simulink library "hvs_framelib_gen"  (R2016a)
settings: Solver=ode45  StartTime=0.0  StopTime=10.0  RelTol=1e-3
undefined symbols (not defined in the file): API4dcac_efficiency, API5dcac_efficiency, aux_power_flag, dcdc_effmap, dcdc_effmap_cooltemp_3rdD, dcdc_effmap_cur_2ndD, dcdc_effmap_vlt_1stD
libraries: Electrical_to_Mechanical_gen x6, Electrical_converter x2, Electrical_to_Thermal_gen x1, Electrical_charger x1, Powernet x1, ePTO x1, simulink x1
settings Model: Creator=krishs1  LastModifiedBy=krishs1
settings DataIOCC: LimitDataPoints=on
settings DebuggingCC: AllowSymbolicDim=off

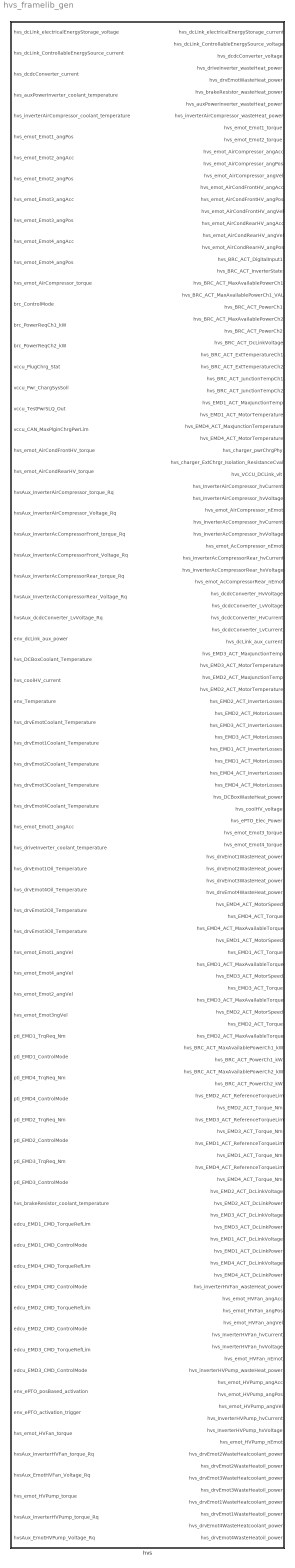
== system hvs_framelib_gen ==
  hvs : Subsystem

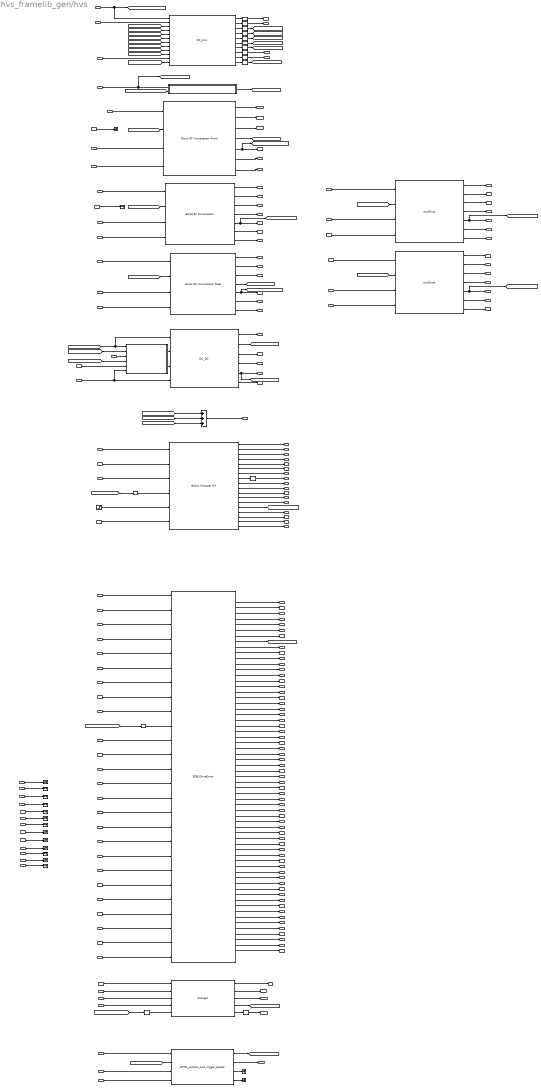
== system hvs_framelib_gen/hvs ==
  hvs_dcLink_electricalEnergyStorage_voltage : Inport
  hvs_dcLink_ControllableEnergySource_current : Inport  Port=2
  hvs_dcdcConverter_current : Inport  Port=3
  hvs_auxPowerInverter_coolant_temperature : Inport  Port=4
  hvs_inverterAirCompressor_coolant_temperature : Inport  Port=5
  hvs_emot_Emot1_angPos : Inport  Port=6
  hvs_emot_Emot2_angAcc : Inport  Port=7
  hvs_emot_Emot2_angPos : Inport  Port=8
  hvs_emot_Emot3_angAcc : Inport  Port=9
  hvs_emot_Emot3_angPos : Inport  Port=10
  hvs_emot_Emot4_angAcc : Inport  Port=11
  hvs_emot_Emot4_angPos : Inport  Port=12
  hvs_emot_AirCompressor_torque : Inport  Port=13
  brc_ControlMode : Inport  Port=14
  brc_PowerReqCh1_kW : Inport  Port=15
  brc_PowerReqCh2_kW : Inport  Port=16
  vccu_PlugChrg_Stat : Inport  Port=17
  vccu_Pwr_ChargSysSoll : Inport  Port=18
  vccu_TestPwrSLQ_Out : Inport  Port=19
  vccu_CAN_MaxPlginChrgPwrLim : Inport  Port=20
  hvs_emot_AirCondFrontHV_torque : Inport  Port=21
  hvs_emot_AirCondRearHV_torque : Inport  Port=22
  hvsAux_InverterAirCompressor_torque_Rq : Inport  Port=23
  hvsAux_InverterAirCompressor_Voltage_Rq : Inport  Port=24
  hvsAux_InverterAcCompressorFront_torque_Rq : Inport  Port=25
  hvsAux_InverterAcCompressorFront_Voltage_Rq : Inport  Port=26
  hvsAux_InverterAcCompressorRear_torque_Rq : Inport  Port=27
  hvsAux_InverterAcCompressorRear_Voltage_Rq : Inport  Port=28
  hvsAux_dcdcConverter_LvVoltage_Rq : Inport  Port=29
  env_dcLink_aux_power : Inport  Port=30
  hvs_DCBoxCoolant_Temperature : Inport  Port=31
  hvs_coolHV_current : Inport  Port=32
  env_Temperature : Inport  Port=33
  hvs_drvEmotCoolant_Temperature : Inport  Port=34
  hvs_drvEmot1Coolant_Temperature : Inport  Port=35
  hvs_drvEmot2Coolant_Temperature : Inport  Port=36
  hvs_drvEmot3Coolant_Temperature : Inport  Port=37
  hvs_drvEmot4Coolant_Temperature : Inport  Port=38
  hvs_emot_Emot1_angAcc : Inport  Port=39
  hvs_driveInverter_coolant_temperature : Inport  Port=40
  hvs_drvEmot1Oil_Temperature : Inport  Port=41
  hvs_drvEmot4Oil_Temperature : Inport  Port=42
  hvs_drvEmot2Oil_Temperature : Inport  Port=43
  hvs_drvEmot3Oil_Temperature : Inport  Port=44
  hvs_emot_Emot1_angVel : Inport  Port=45
  hvs_emot_Emot4_angVel : Inport  Port=46
  hvs_emot_Emot2_angVel : Inport  Port=47
  hvs_emot_Emot3ngVel : Inport  Port=48
  pti_EMD1_TrqReq_Nm : Inport  Port=49
  pti_EMD1_ControlMode : Inport  Port=50
  pti_EMD4_TrqReq_Nm : Inport  Port=51
  pti_EMD4_ControlMode : Inport  Port=52
  pti_EMD2_TrqReq_Nm : Inport  Port=53
  pti_EMD2_ControlMode : Inport  Port=54
  pti_EMD3_TrqReq_Nm : Inport  Port=55
  pti_EMD3_ControlMode : Inport  Port=56
  hvs_brakeResistor_coolant_temperature : Inport  Port=57
  edcu_EMD1_CMD_TorqueRefLim : Inport  Port=58
  edcu_EMD1_CMD_ControlMode : Inport  Port=59
  edcu_EMD4_CMD_TorqueRefLim : Inport  Port=60
  edcu_EMD4_CMD_ControlMode : Inport  Port=61
  edcu_EMD2_CMD_TorqueRefLim : Inport  Port=62
  edcu_EMD2_CMD_ControlMode : Inport  Port=63
  edcu_EMD3_CMD_TorqueRefLim : Inport  Port=64
  edcu_EMD3_CMD_ControlMode : Inport  Port=65
  env_ePTO_posBased_activation : Inport  Port=66
  env_ePTO_activation_trigger : Inport  Port=67
  hvs_emot_HVFan_torque : Inport  Port=68
  hvsAux_InverterHVFan_torque_Rq : Inport  Port=69
  hvsAux_EmotHVFan_Voltage_Rq : Inport  Port=70
  hvs_emot_HVPump_torque : Inport  Port=71
  hvsAux_InverterHVPump_torque_Rq : Inport  Port=72
  hvsAux_EmotHVPump_Voltage_Rq : Inport  Port=73
  Brake Chopper RX : Electrical_to_Thermal_gen/Brake Chopper RX
  Charger : Electrical_charger/Charger
  DC_DC : Electrical_converter/DC_DC
  DC_Link : Powernet/DC_Link
  EDB_DriveEmot : Electrical_to_Mechanical_gen/EDB_DriveEmot
  Emot AC Compressor Front : Electrical_to_Mechanical_gen/Emot AC Compressor Front
  Emot AC Compressor Rear : Electrical_to_Mechanical_gen/Emot AC Compressor Rear
  Emot Air Compressor : Electrical_to_Mechanical_gen/Emot Air Compressor
  Emotor Hv Fan : Electrical_to_Mechanical_gen/auxEmot  auxEmot_nTab_3rdD=emot_HVFan_nTab_3rdD  auxEmot_trqTab_2ndD=emot_HVFan_trqTab_2ndD  auxEmot_vltTab_1stD=emot_HVFan_vltTab_1stD  auxEmot_pwrAC=emot_HVFan_pwrAC  APIefficiency=1/API4dcac_efficiency  auxEmot_inertia=emot_HVFan_inertia  auxEmot_Tau=emot_HVFan_Tau  AWR_InvStError=0  auxEmot_power=0  aux_power_state=0
  Emotor Hv Pump : Electrical_to_Mechanical_gen/auxEmot  auxEmot_nTab_3rdD=emot_HVPump_nTab_3rdD  auxEmot_trqTab_2ndD=emot_HVPump_trqTab_2ndD  auxEmot_vltTab_1stD=emot_HVPump_vltTab_1stD  auxEmot_pwrAC=emot_HVPump_pwrAC  APIefficiency=1/API5dcac_efficiency  auxEmot_inertia=emot_HVPump_inertia  auxEmot_Tau=emot_HVPump_Tau  AWR_InvStError=0  auxEmot_power=0  aux_power_state=0
  HVFreigabeHW2_SiRelay_D : Step  Time=5.502
  Process : Subsystem
  Reshape{,1..8,11..12,14..17} (15 alike) : Reshape
  Sum8 : Sum  Inputs=+++  SaturateOnIntegerOverflow=on  InputSameDT=on  OutDataTypeStr=Inherit: Same as first input
  Terminator{,1..16} (17 alike) : Terminator
  ePTO_position_and_trigger_based : ePTO/ePTO_position_and_trigger_based
  sub_env_aux : Subsystem
  hvs_dcLink_electricalEnergyStorage_current : Outport
  hvs_dcLink_ControllableEnergySource_voltage : Outport  Port=2
  hvs_dcdcConverter_voltage : Outport  Port=3
  hvs_driveInverter_wasteHeat_power : Outport  Port=4
  hvs_drvEmotWasteHeat_power : Outport  Port=5
  hvs_brakeResistor_wasteHeat_power : Outport  Port=6
  hvs_auxPowerInverter_wasteHeat_power : Outport  Port=7
  hvs_inverterAirCompressor_wasteHeat_power : Outport  Port=8
  hvs_emot_Emot1_torque : Outport  Port=9
  hvs_emot_Emot2_torque : Outport  Port=10
  hvs_emot_AirCompressor_angAcc : Outport  Port=11
  hvs_emot_AirCompressor_angPos : Outport  Port=12
  hvs_emot_AirCompressor_angVel : Outport  Port=13
  hvs_emot_AirCondFrontHV_angAcc : Outport  Port=14
  hvs_emot_AirCondFrontHV_angPos : Outport  Port=15
  hvs_emot_AirCondFrontHV_angVel : Outport  Port=16
  hvs_emot_AirCondRearHV_angAcc : Outport  Port=17
  hvs_emot_AirCondRearHV_angVel : Outport  Port=18
  hvs_emot_AirCondRearHV_angPos : Outport  Port=19
  hvs_BRC_ACT_DigitalInput1 : Outport  Port=20
  hvs_BRC_ACT_InverterState : Outport  Port=21
  hvs_BRC_ACT_MaxAvailablePowerCh1 : Outport  Port=22
  hvs_BRC_ACT_MaxAvailablePowerCh1_VAL : Outport  Port=23
  hvs_BRC_ACT_PowerCh1 : Outport  Port=24
  hvs_BRC_ACT_MaxAvailablePowerCh2 : Outport  Port=25
  hvs_BRC_ACT_PowerCh2 : Outport  Port=26
  hvs_BRC_ACT_DcLinkVoltage : Outport  Port=27
  hvs_BRC_ACT_ExtTemperatureCh1 : Outport  Port=28
  hvs_BRC_ACT_ExtTemperatureCh2 : Outport  Port=29
  hvs_BRC_ACT_JunctionTempCh1 : Outport  Port=30
  hvs_BRC_ACT_JunctionTempCh2 : Outport  Port=31
  hvs_EMD1_ACT_MaxJunctionTemp : Outport  Port=32
  hvs_EMD1_ACT_MotorTemperature : Outport  Port=33
  hvs_EMD4_ACT_MaxJunctionTemperature : Outport  Port=34
  hvs_EMD4_ACT_MotorTemperature : Outport  Port=35
  hvs_charger_pwrChrgPhy : Outport  Port=36
  hvs_charger_ExtChrgr_Isolation_ResistanceCval : Outport  Port=37
  hvs_VCCU_DCLink_vlt : Outport  Port=38
  hvs_InverterAirCompressor_hvCurrent : Outport  Port=39
  hvs_InverterAirCompressor_hvVoltage : Outport  Port=40
  hvs_emot_AirCompressor_nEmot : Outport  Port=41
  hvs_InverterAcCompressor_hvCurrent : Outport  Port=42
  hvs_InverterAcCompressor_hvVoltage : Outport  Port=43
  hvs_emot_AcCompressor_nEmot : Outport  Port=44
  hvs_InverterAcCompressorRear_hvCurrent : Outport  Port=45
  hvs_InverterAcCompressorRear_hvVoltage : Outport  Port=46
  hvs_emot_AcCompressorRear_nEmot : Outport  Port=47
  hvs_dcdcConverter_HvVoltage : Outport  Port=48
  hvs_dcdcConverter_LvVoltage : Outport  Port=49
  hvs_dcdcConverter_HvCurrent : Outport  Port=50
  hvs_dcdcConverter_LvCurrent : Outport  Port=51
  hvs_dcLink_aux_current : Outport  Port=52
  hvs_EMD3_ACT_MaxJunctionTemp : Outport  Port=53
  hvs_EMD3_ACT_MotorTemperature : Outport  Port=54
  hvs_EMD2_ACT_MaxJunctionTemp : Outport  Port=55
  hvs_EMD2_ACT_MotorTemperature : Outport  Port=56
  hvs_EMD2_ACT_InverterLosses : Outport  Port=57
  hvs_EMD2_ACT_MotorLosses : Outport  Port=58
  hvs_EMD3_ACT_InverterLosses : Outport  Port=59
  hvs_EMD3_ACT_MotorLosses : Outport  Port=60
  hvs_EMD1_ACT_InverterLosses : Outport  Port=61
  hvs_EMD1_ACT_MotorLosses : Outport  Port=62
  hvs_EMD4_ACT_InverterLosses : Outport  Port=63
  hvs_EMD4_ACT_MotorLosses : Outport  Port=64
  hvs_DCBoxWasteHeat_power : Outport  Port=65
  hvs_coolHV_voltage : Outport  Port=66
  hvs_ePTO_Elec_Power : Outport  Port=67
  hvs_emot_Emot3_torque : Outport  Port=68
  hvs_emot_Emot4_torque : Outport  Port=69
  hvs_drvEmot1WasteHeat_power : Outport  Port=70
  hvs_drvEmot2WasteHeat_power : Outport  Port=71
  hvs_drvEmot3WasteHeat_power : Outport  Port=72
  hvs_drvEmot4WasteHeat_power : Outport  Port=73
  hvs_EMD4_ACT_MotorSpeed : Outport  Port=74
  hvs_EMD4_ACT_Torque : Outport  Port=75
  hvs_EMD4_ACT_MaxAvailableTorque : Outport  Port=76
  hvs_EMD1_ACT_MotorSpeed : Outport  Port=77
  hvs_EMD1_ACT_Torque : Outport  Port=78
  hvs_EMD1_ACT_MaxAvailableTorque : Outport  Port=79
  hvs_EMD3_ACT_MotorSpeed : Outport  Port=80
  hvs_EMD3_ACT_Torque : Outport  Port=81
  hvs_EMD3_ACT_MaxAvailableTorque : Outport  Port=82
  hvs_EMD2_ACT_MotorSpeed : Outport  Port=83
  hvs_EMD2_ACT_Torque : Outport  Port=84
  hvs_EMD2_ACT_MaxAvailableTorque : Outport  Port=85
  hvs_BRC_ACT_MaxAvailablePowerCh1_kW : Outport  Port=86
  hvs_BRC_ACT_PowerCh1_kW : Outport  Port=87
  hvs_BRC_ACT_MaxAvailablePowerCh2_kW : Outport  Port=88
  hvs_BRC_ACT_PowerCh2_kW : Outport  Port=89
  hvs_EMD2_ACT_ReferenceTorqueLim : Outport  Port=90
  hvs_EMD2_ACT_Torque_Nm : Outport  Port=91
  hvs_EMD3_ACT_ReferenceTorqueLim : Outport  Port=92
  hvs_EMD3_ACT_Torque_Nm : Outport  Port=93
  hvs_EMD1_ACT_ReferenceTorqueLim : Outport  Port=94
  hvs_EMD1_ACT_Torque_Nm : Outport  Port=95
  hvs_EMD4_ACT_ReferenceTorqueLim : Outport  Port=96
  hvs_EMD4_ACT_Torque_Nm : Outport  Port=97
  hvs_EMD2_ACT_DcLinkVoltage : Outport  Port=98
  hvs_EMD2_ACT_DcLinkPower : Outport  Port=99
  hvs_EMD3_ACT_DcLinkVoltage : Outport  Port=100
  hvs_EMD3_ACT_DcLinkPower : Outport  Port=101
  hvs_EMD1_ACT_DcLinkVoltage : Outport  Port=102
  hvs_EMD1_ACT_DcLinkPower : Outport  Port=103
  hvs_EMD4_ACT_DcLinkVoltage : Outport  Port=104
  hvs_EMD4_ACT_DcLinkPower : Outport  Port=105
  hvs_inverterHVFan_wasteHeat_power : Outport  Port=106
  hvs_emot_HVFan_angAcc : Outport  Port=107
  hvs_emot_HVFan_angPos : Outport  Port=108
  hvs_emot_HVFan_angVel : Outport  Port=109
  hvs_InverterHVFan_hvCurrent : Outport  Port=110
  hvs_InverterHVFan_hvVoltage : Outport  Port=111
  hvs_emot_HVFan_nEmot : Outport  Port=112
  hvs_inverterHVPump_wasteHeat_power : Outport  Port=113
  hvs_emot_HVPump_angAcc : Outport  Port=114
  hvs_emot_HVPump_angPos : Outport  Port=115
  hvs_emot_HVPump_angVel : Outport  Port=116
  hvs_InverterHVPump_hvCurrent : Outport  Port=117
  hvs_InverterHVPump_hvVoltage : Outport  Port=118
  hvs_emot_HVPump_nEmot : Outport  Port=119
  hvs_drvEmot2WasteHeatcoolant_power : Outport  Port=120
  hvs_drvEmot2WasteHeatoil_power : Outport  Port=121
  hvs_drvEmot3WasteHeatcoolant_power : Outport  Port=122
  hvs_drvEmot3WasteHeatoil_power : Outport  Port=123
  hvs_drvEmot1WasteHeatcoolant_power : Outport  Port=124
  hvs_drvEmot1WasteHeatoil_power : Outport  Port=125
  hvs_drvEmot4WasteHeatcoolant_power : Outport  Port=126
  hvs_drvEmot4WasteHeatoil_power : Outport  Port=127
  wires:
  EDB_DriveEmot/29 -> hvs_EMD4_ACT_Torque/1
  EDB_DriveEmot/28 -> hvs_EMD4_ACT_MotorSpeed/1
  EDB_DriveEmot/27 -> hvs_drvEmot4WasteHeat_power/1
  EDB_DriveEmot/26 -> hvs_drvEmot3WasteHeat_power/1
  EDB_DriveEmot/8 -> [hvs_dcLink_drive_emot_current]
  hvs_drvEmot4Coolant_Temperature/1 -> Terminator14/1
  hvs_drvEmot3Coolant_Temperature/1 -> Terminator13/1
  hvs_drvEmot2Coolant_Temperature/1 -> Terminator12/1
  hvs_drvEmot1Coolant_Temperature/1 -> Terminator11/1
  EDB_DriveEmot/25 -> hvs_drvEmot2WasteHeat_power/1
  EDB_DriveEmot/24 -> hvs_drvEmot1WasteHeat_power/1
  hvs_emot_Emot4_angPos/1 -> Terminator10/1
  hvs_emot_Emot4_angAcc/1 -> Terminator9/1
  hvs_emot_Emot3_angPos/1 -> Terminator8/1
  hvs_emot_Emot3_angAcc/1 -> Terminator6/1
  Process/2(hvs_dcdcConv_current1) -> DC_DC/3
  Process/1(dcdc_conv_eff) -> DC_DC/2
  hvs_dcdcConverter_current/1 -> Process/5(hvs_dcdcConv_current)
  [dcLink_aux_power] -> Process/4(dcLink_aux_power)  "dcLink_aux_power"
  hvs_drvEmotCoolant_Temperature/1 -> Process/3(hvs_drvEmotCoolant_Temperature)
  [hvs_dcdc_current] -> Process/2(hvs_dcdc_HvCurrent)  "hvs_dcdc_HvCurrent"
  [hvs_dcLink_ePTO_current] -> DC_Link/12
  [hvs_APIs_DCLink_vlt] -> ePTO_position_and_trigger_based/2
  ePTO_position_and_trigger_based/3 -> Terminator7/1
  ePTO_position_and_trigger_based/2 -> hvs_ePTO_Elec_Power/1
  ePTO_position_and_trigger_based/1 -> [hvs_dcLink_ePTO_current]
  DC_Link/10 -> Reshape17/1
  Reshape17/1 -> [hvs_ePTO_DCLink_vlt]
  env_Temperature/1 -> ePTO_position_and_trigger_based/1
  EDB_DriveEmot/23 -> hvs_emot_Emot4_torque/1
  EDB_DriveEmot/22 -> hvs_emot_Emot3_torque/1
  hvs_DCBoxCoolant_Temperature/1 -> Terminator4/1
  Charger/1 -> hvs_DCBoxWasteHeat_power/1  "hvs_DCBoxWasteHeat_power"
  hvsAux_dcdcConverter_LvVoltage_Rq/1 -> DC_DC/4, Process/6(hvsAux_dcdcConv_LvVoltage_Rq)  "hvsAux_dcdcConverter_LvVoltage_Rq"
  DC_Link/8 -> Reshape15/1
  [hvs_dcLink_electricalEnergyStorage_voltage] -> sub_env_aux/2(Nebenagg_voltage)
  sub_env_aux/1(dcLink_aux_current) -> [dcLink_aux_current]
  env_dcLink_aux_power/1 -> sub_env_aux/1(env_dcLink_aux_power), [dcLink_aux_power]
  [dcLink_aux_current] -> DC_Link/10
  Reshape12/1 -> hvs_VCCU_DCLink_vlt/1
  Reshape11/1 -> Charger/5
  Reshape7/1 -> hvs_BRC_ACT_DcLinkVoltage/1
  Reshape6/1 -> Brake Chopper RX/4
  Reshape5/1 -> [hvs_APIs_DCLink_vlt]
  Reshape4/1 -> [hvs_charger_DCLink_vlt]
  Reshape3/1 -> [hvs_inverter_drive_emot_voltage]
  Reshape2/1 -> [hvs_inverter_BrakeResistor_voltage]
  Reshape1/1 -> [hvs_dcdcConverter_voltage]
  Reshape/1 -> hvs_dcLink_electricalEnergyStorage_current/1
  [hvs_dcdc_current] -> DC_Link/3
  [hvs_DCL_wasteHeat_power] -> Sum8/3
  [hvs_API3_wasteHeat_power] -> Sum8/2
  [hvs_API1_wasteHeat_power] -> Sum8/1
  Sum8/1 -> hvs_auxPowerInverter_wasteHeat_power/1
  DC_DC/6 -> hvs_dcdcConverter_LvCurrent/1
  DC_DC/5 -> hvs_dcdcConverter_HvCurrent/1, [hvs_dcdc_current]
  DC_DC/4 -> hvs_dcdcConverter_LvVoltage/1
  DC_DC/3 -> hvs_dcdcConverter_HvVoltage/1
  DC_Link/3 -> Reshape1/1
  DC_DC/1 -> hvs_dcdcConverter_voltage/1
  DC_DC/2 -> [hvs_DCL_wasteHeat_power]
  [hvs_dcdcConverter_voltage] -> Process/1(hvs_dcdcConverter_voltage), DC_DC/1  "hvs_dcdcConverter_voltage"
  Emot AC Compressor Rear/4 -> [hvs_API3_wasteHeat_power]
  Emot AC Compressor Rear/5 -> hvs_InverterAcCompressorRear_hvCurrent/1, [hvs_InverterAcCompressorRear_hvCurrent]
  Emot AC Compressor Rear/6 -> hvs_InverterAcCompressorRear_hvVoltage/1
  Emot AC Compressor Rear/7 -> hvs_emot_AcCompressorRear_nEmot/1
  Emot AC Compressor Rear/2 -> hvs_emot_AirCondRearHV_angPos/1
  Emot AC Compressor Rear/3 -> hvs_emot_AirCondRearHV_angVel/1
  Emot AC Compressor Rear/1 -> hvs_emot_AirCondRearHV_angAcc/1
  hvsAux_InverterAcCompressorRear_Voltage_Rq/1 -> Emot AC Compressor Rear/4
  hvsAux_InverterAcCompressorRear_torque_Rq/1 -> Emot AC Compressor Rear/3
  [hvs_APIs_DCLink_vlt] -> Emot AC Compressor Rear/2
  hvs_emot_AirCondRearHV_torque/1 -> Emot AC Compressor Rear/1
  Emot AC Compressor Front/4 -> [hvs_API1_wasteHeat_power]
  Emot AC Compressor Front/6 -> hvs_InverterAcCompressor_hvVoltage/1
  Emot AC Compressor Front/7 -> hvs_emot_AcCompressor_nEmot/1
  Emot AC Compressor Front/3 -> hvs_emot_AirCondFrontHV_angVel/1
  Emot AC Compressor Front/2 -> hvs_emot_AirCondFrontHV_angPos/1
  Emot AC Compressor Front/1 -> hvs_emot_AirCondFrontHV_angAcc/1
  hvsAux_InverterAcCompressorFront_Voltage_Rq/1 -> Emot AC Compressor Front/4
  hvsAux_InverterAcCompressorFront_torque_Rq/1 -> Emot AC Compressor Front/3
  hvs_emot_AirCondFrontHV_torque/1 -> Emot AC Compressor Front/1
  [hvs_APIs_DCLink_vlt] -> Emot AC Compressor Front/2
  hvs_auxPowerInverter_coolant_temperature/1 -> Terminator5/1
  hvs_inverterAirCompressor_coolant_temperature/1 -> Terminator/1
  hvsAux_InverterAirCompressor_Voltage_Rq/1 -> Emot Air Compressor/4
  hvsAux_InverterAirCompressor_torque_Rq/1 -> Emot Air Compressor/3
  [hvs_APIs_DCLink_vlt] -> Emot Air Compressor/2
  DC_Link/7 -> Reshape5/1
  Emot Air Compressor/6 -> hvs_InverterAirCompressor_hvVoltage/1
  Emot Air Compressor/7 -> hvs_emot_AirCompressor_nEmot/1
  Emot Air Compressor/5 -> [hvs_emot_AirCompressor_emot_current], hvs_InverterAirCompressor_hvCurrent/1
  Emot Air Compressor/4 -> hvs_inverterAirCompressor_wasteHeat_power/1
  Emot Air Compressor/3 -> hvs_emot_AirCompressor_angVel/1
  Emot Air Compressor/2 -> hvs_emot_AirCompressor_angPos/1
  Emot Air Compressor/1 -> hvs_emot_AirCompressor_angAcc/1
  hvs_emot_AirCompressor_torque/1 -> Emot Air Compressor/1
  DC_Link/1 -> Reshape/1
  DC_Link/2 -> Reshape14/1
  hvs_dcLink_electricalEnergyStorage_voltage/1 -> [hvs_dcLink_electricalEnergyStorage_voltage], DC_Link/1
  hvs_dcLink_ControllableEnergySource_current/1 -> DC_Link/2
  DC_Link/4 -> Reshape2/1
  Brake Chopper RX/1 -> hvs_BRC_ACT_DigitalInput1/1
  Brake Chopper RX/2 -> hvs_BRC_ACT_InverterState/1
  Brake Chopper RX/3 -> hvs_BRC_ACT_MaxAvailablePowerCh1/1
  Brake Chopper RX/4 -> hvs_BRC_ACT_MaxAvailablePowerCh1_VAL/1
  Brake Chopper RX/5 -> hvs_BRC_ACT_PowerCh1/1
  Brake Chopper RX/6 -> hvs_BRC_ACT_MaxAvailablePowerCh2/1
  Brake Chopper RX/7 -> hvs_BRC_ACT_PowerCh2/1
  Brake Chopper RX/8 -> Reshape7/1
  Brake Chopper RX/9 -> hvs_BRC_ACT_ExtTemperatureCh1/1
  Brake Chopper RX/10 -> hvs_BRC_ACT_ExtTemperatureCh2/1
  Brake Chopper RX/11 -> hvs_BRC_ACT_JunctionTempCh1/1
  Brake Chopper RX/12 -> hvs_BRC_ACT_JunctionTempCh2/1
  [hvs_inverter_BrakeResistor_voltage] -> Reshape6/1
  DC_Link/5 -> Reshape3/1
  [hvs_dcLink_drive_emot_current] -> DC_Link/4
  [hvs_emot_AirCompressor_emot_current] -> DC_Link/5
  Brake Chopper RX/13 -> hvs_brakeResistor_wasteHeat_power/1
  Brake Chopper RX/14 -> [hvs_dcLink_BrakeResistor_current]
  [hvs_dcLink_BrakeResistor_current] -> DC_Link/6
  hvs_emot_Emot1_angPos/1 -> Terminator1/1
  hvs_emot_Emot2_angAcc/1 -> Terminator2/1
  hvs_emot_Emot2_angPos/1 -> Terminator3/1
  EDB_DriveEmot/13 -> hvs_emot_Emot2_torque/1
  EDB_DriveEmot/4 -> hvs_EMD1_ACT_MaxJunctionTemp/1
  EDB_DriveEmot/5 -> hvs_EMD1_ACT_MotorTemperature/1
  EDB_DriveEmot/6 -> hvs_EMD4_ACT_MaxJunctionTemperature/1
  EDB_DriveEmot/7 -> hvs_EMD4_ACT_MotorTemperature/1
  vccu_CAN_MaxPlginChrgPwrLim/1 -> Charger/4
  [hvs_charger_DCLink_vlt] -> Reshape11/1
  vccu_TestPwrSLQ_Out/1 -> Charger/3
  vccu_Pwr_ChargSysSoll/1 -> Charger/2
  vccu_PlugChrg_Stat/1 -> Charger/1
  Charger/2 -> hvs_charger_pwrChrgPhy/1
  Charger/3 -> hvs_charger_ExtChrgr_Isolation_ResistanceCval/1
  Charger/4 -> [hvs_dcLink_charger_current]
  [hvs_dcLink_charger_current] -> DC_Link/7
  DC_Link/6 -> Reshape4/1
  Charger/5 -> Reshape12/1
  Emot AC Compressor Front/5 -> [hvs_InverterAcCompressor_hvCurrent], hvs_InverterAcCompressor_hvCurrent/1
  [hvs_InverterAcCompressor_hvCurrent] -> DC_Link/8
  [hvs_InverterAcCompressorRear_hvCurrent] -> DC_Link/9
  EDB_DriveEmot/1 -> hvs_emot_Emot1_torque/1
  EDB_DriveEmot/2 -> hvs_driveInverter_wasteHeat_power/1
  EDB_DriveEmot/3 -> hvs_drvEmotWasteHeat_power/1
  EDB_DriveEmot/9 -> hvs_EMD3_ACT_MaxJunctionTemp/1
  EDB_DriveEmot/10 -> hvs_EMD3_ACT_MotorTemperature/1
  EDB_DriveEmot/11 -> hvs_EMD2_ACT_MaxJunctionTemp/1
  EDB_DriveEmot/12 -> hvs_EMD2_ACT_MotorTemperature/1
  EDB_DriveEmot/14 -> hvs_EMD2_ACT_InverterLosses/1
  EDB_DriveEmot/15 -> hvs_EMD2_ACT_MotorLosses/1
  EDB_DriveEmot/16 -> hvs_EMD3_ACT_InverterLosses/1
  EDB_DriveEmot/17 -> hvs_EMD3_ACT_MotorLosses/1
  EDB_DriveEmot/18 -> hvs_EMD1_ACT_InverterLosses/1
  EDB_DriveEmot/19 -> hvs_EMD1_ACT_MotorLosses/1
  EDB_DriveEmot/20 -> hvs_EMD4_ACT_InverterLosses/1
  EDB_DriveEmot/21 -> hvs_EMD4_ACT_MotorLosses/1
  Reshape14/1 -> hvs_dcLink_ControllableEnergySource_voltage/1
  Reshape15/1 -> hvs_dcLink_aux_current/1
  DC_Link/9 -> Reshape16/1
  Reshape16/1 -> hvs_coolHV_voltage/1
  hvs_coolHV_current/1 -> DC_Link/11
  hvs_emot_Emot1_angAcc/1 -> Terminator15/1
  EDB_DriveEmot/30 -> hvs_EMD4_ACT_MaxAvailableTorque/1
  EDB_DriveEmot/31 -> hvs_EMD1_ACT_MotorSpeed/1
  EDB_DriveEmot/32 -> hvs_EMD1_ACT_Torque/1
  EDB_DriveEmot/33 -> hvs_EMD1_ACT_MaxAvailableTorque/1
  EDB_DriveEmot/34 -> hvs_EMD3_ACT_MotorSpeed/1
  EDB_DriveEmot/35 -> hvs_EMD3_ACT_Torque/1
  EDB_DriveEmot/36 -> hvs_EMD3_ACT_MaxAvailableTorque/1
  EDB_DriveEmot/37 -> hvs_EMD2_ACT_MotorSpeed/1
  EDB_DriveEmot/38 -> hvs_EMD2_ACT_Torque/1
  EDB_DriveEmot/39 -> hvs_EMD2_ACT_MaxAvailableTorque/1
  EDB_DriveEmot/40 -> hvs_EMD2_ACT_ReferenceTorqueLim/1
  EDB_DriveEmot/41 -> hvs_EMD2_ACT_Torque_Nm/1
  hvs_driveInverter_coolant_temperature/1 -> EDB_DriveEmot/1
  hvs_drvEmot1Oil_Temperature/1 -> EDB_DriveEmot/2
  hvs_drvEmot4Oil_Temperature/1 -> EDB_DriveEmot/3
  hvs_drvEmot2Oil_Temperature/1 -> EDB_DriveEmot/4
  hvs_drvEmot3Oil_Temperature/1 -> EDB_DriveEmot/5
  hvs_emot_Emot1_angVel/1 -> EDB_DriveEmot/6
  hvs_emot_Emot4_angVel/1 -> EDB_DriveEmot/7
  hvs_emot_Emot2_angVel/1 -> EDB_DriveEmot/8
  hvs_emot_Emot3ngVel/1 -> EDB_DriveEmot/9
  [hvs_inverter_drive_emot_voltage] -> Reshape8/1
  Reshape8/1 -> EDB_DriveEmot/10
  HVFreigabeHW2_SiRelay_D/1 -> Brake Chopper RX/5
  pti_EMD1_TrqReq_Nm/1 -> EDB_DriveEmot/11
  pti_EMD1_ControlMode/1 -> EDB_DriveEmot/12
  pti_EMD4_TrqReq_Nm/1 -> EDB_DriveEmot/13
  pti_EMD4_ControlMode/1 -> EDB_DriveEmot/14
  pti_EMD2_TrqReq_Nm/1 -> EDB_DriveEmot/15
  pti_EMD2_ControlMode/1 -> EDB_DriveEmot/16
  pti_EMD3_TrqReq_Nm/1 -> EDB_DriveEmot/17
  pti_EMD3_ControlMode/1 -> EDB_DriveEmot/18
  brc_ControlMode/1 -> Brake Chopper RX/1
  brc_PowerReqCh1_kW/1 -> Brake Chopper RX/2
  brc_PowerReqCh2_kW/1 -> Brake Chopper RX/3
  hvs_brakeResistor_coolant_temperature/1 -> Brake Chopper RX/6
  Brake Chopper RX/15 -> hvs_BRC_ACT_MaxAvailablePowerCh1_kW/1
  Brake Chopper RX/16 -> hvs_BRC_ACT_PowerCh1_kW/1
  Brake Chopper RX/17 -> hvs_BRC_ACT_MaxAvailablePowerCh2_kW/1
  Brake Chopper RX/18 -> hvs_BRC_ACT_PowerCh2_kW/1
  EDB_DriveEmot/42 -> hvs_EMD3_ACT_ReferenceTorqueLim/1
  EDB_DriveEmot/44 -> hvs_EMD1_ACT_ReferenceTorqueLim/1
  EDB_DriveEmot/46 -> hvs_EMD4_ACT_ReferenceTorqueLim/1
  EDB_DriveEmot/47 -> hvs_EMD4_ACT_Torque_Nm/1
  EDB_DriveEmot/45 -> hvs_EMD1_ACT_Torque_Nm/1
  EDB_DriveEmot/48 -> hvs_EMD2_ACT_DcLinkVoltage/1
  EDB_DriveEmot/49 -> hvs_EMD2_ACT_DcLinkPower/1
  EDB_DriveEmot/50 -> hvs_EMD3_ACT_DcLinkVoltage/1
  EDB_DriveEmot/51 -> hvs_EMD3_ACT_DcLinkPower/1
  EDB_DriveEmot/52 -> hvs_EMD1_ACT_DcLinkVoltage/1
  EDB_DriveEmot/43 -> hvs_EMD3_ACT_Torque_Nm/1
  EDB_DriveEmot/54 -> hvs_EMD4_ACT_DcLinkVoltage/1
  EDB_DriveEmot/55 -> hvs_EMD4_ACT_DcLinkPower/1
  EDB_DriveEmot/53 -> hvs_EMD1_ACT_DcLinkPower/1
  edcu_EMD4_CMD_ControlMode/1 -> EDB_DriveEmot/22
  edcu_EMD2_CMD_ControlMode/1 -> EDB_DriveEmot/24
  edcu_EMD2_CMD_TorqueRefLim/1 -> EDB_DriveEmot/23
  edcu_EMD3_CMD_ControlMode/1 -> EDB_DriveEmot/26
  edcu_EMD3_CMD_TorqueRefLim/1 -> EDB_DriveEmot/25
  edcu_EMD4_CMD_TorqueRefLim/1 -> EDB_DriveEmot/21
  edcu_EMD1_CMD_TorqueRefLim/1 -> EDB_DriveEmot/19
  edcu_EMD1_CMD_ControlMode/1 -> EDB_DriveEmot/20
  ePTO_position_and_trigger_based/4 -> Terminator16/1
  env_ePTO_posBased_activation/1 -> ePTO_position_and_trigger_based/3
  env_ePTO_activation_trigger/1 -> ePTO_position_and_trigger_based/4
  hvsAux_EmotHVFan_Voltage_Rq/1 -> Emotor Hv Fan/4
  hvsAux_InverterHVFan_torque_Rq/1 -> Emotor Hv Fan/3
  [hvs_APIs_DCLink_vlt] -> Emotor Hv Fan/2
  Emotor Hv Fan/6 -> hvs_InverterHVFan_hvVoltage/1
  Emotor Hv Fan/7 -> hvs_emot_HVFan_nEmot/1
  Emotor Hv Fan/5 -> [hvs_emot_HVFan_emot_current], hvs_InverterHVFan_hvCurrent/1
  Emotor Hv Fan/4 -> hvs_inverterHVFan_wasteHeat_power/1
  Emotor Hv Fan/3 -> hvs_emot_HVFan_angVel/1
  Emotor Hv Fan/2 -> hvs_emot_HVFan_angPos/1
  Emotor Hv Fan/1 -> hvs_emot_HVFan_angAcc/1
  hvs_emot_HVFan_torque/1 -> Emotor Hv Fan/1
  [hvs_APIs_DCLink_vlt] -> Emotor Hv Pump/2
  hvsAux_EmotHVPump_Voltage_Rq/1 -> Emotor Hv Pump/4
  hvsAux_InverterHVPump_torque_Rq/1 -> Emotor Hv Pump/3
  hvs_emot_HVPump_torque/1 -> Emotor Hv Pump/1
  Emotor Hv Pump/6 -> hvs_InverterHVPump_hvVoltage/1
  Emotor Hv Pump/7 -> hvs_emot_HVPump_nEmot/1
  Emotor Hv Pump/5 -> [hvs_emot_HVPump_emot_current], hvs_InverterHVPump_hvCurrent/1
  Emotor Hv Pump/4 -> hvs_inverterHVPump_wasteHeat_power/1
  Emotor Hv Pump/3 -> hvs_emot_HVPump_angVel/1
  Emotor Hv Pump/2 -> hvs_emot_HVPump_angPos/1
  Emotor Hv Pump/1 -> hvs_emot_HVPump_angAcc/1
  EDB_DriveEmot/56 -> hvs_drvEmot2WasteHeatcoolant_power/1
  EDB_DriveEmot/57 -> hvs_drvEmot2WasteHeatoil_power/1
  EDB_DriveEmot/58 -> hvs_drvEmot3WasteHeatcoolant_power/1
  EDB_DriveEmot/59 -> hvs_drvEmot3WasteHeatoil_power/1
  EDB_DriveEmot/60 -> hvs_drvEmot1WasteHeatcoolant_power/1
  EDB_DriveEmot/61 -> hvs_drvEmot1WasteHeatoil_power/1
  EDB_DriveEmot/63 -> hvs_drvEmot4WasteHeatoil_power/1
  EDB_DriveEmot/62 -> hvs_drvEmot4WasteHeatcoolant_power/1

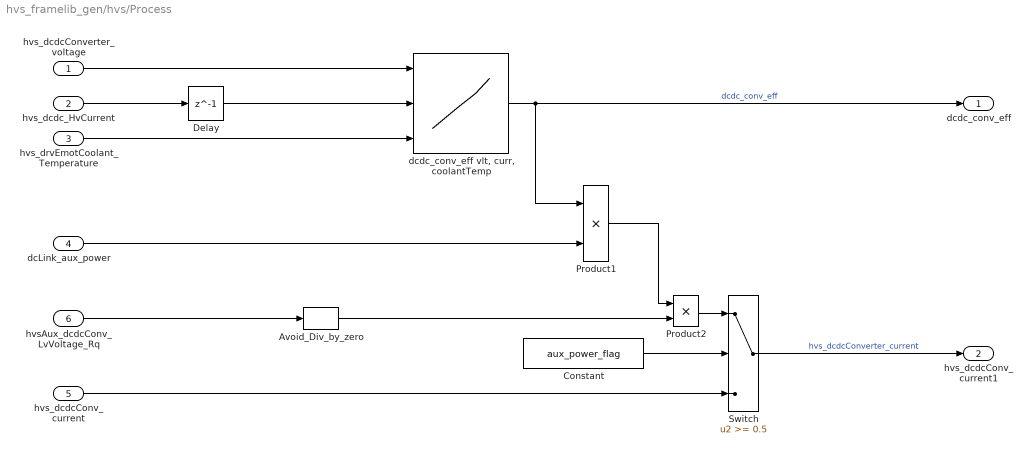
== system hvs_framelib_gen/hvs/Process ==
  hvs_dcdcConverter_voltage : Inport
  hvs_dcdc_HvCurrent : Inport  Port=2
  hvs_drvEmotCoolant_Temperature : Inport  Port=3
  dcLink_aux_power : Inport  Port=4
  hvs_dcdcConv_current : Inport  Port=5
  hvsAux_dcdcConv_LvVoltage_Rq : Inport  Port=6
  Avoid_Div_by_zero : Electrical_converter/DC_DC/Avoid_Div_by_zero
  Constant : Constant  Value=aux_power_flag
  Delay : Delay  DelayLength=1  InitialCondition=0
  Product1 : Product  Inputs=**  RndMeth=Zero
  Product2 : Product  Inputs=**  RndMeth=Zero
  Switch : Switch  Threshold=0.5
  "dcdc_conv_eff vlt, curr, coolantTemp" : Lookup_n-D  NumberOfTableDimensions=3  BreakpointsForDimension1=dcdc_effmap_vlt_1stD  BreakpointsForDimension2=dcdc_effmap_cur_2ndD  BreakpointsForDimension3=dcdc_effmap_cooltemp_3rdD  Table=dcdc_effmap  ExtrapMethod=Clip  RndMeth=Simplest  InputSameDT=on
  dcdc_conv_eff : Outport
  hvs_dcdcConv_current1 : Outport  Port=2
  wires:
  Delay/1 -> "dcdc_conv_eff vlt, curr, coolantTemp"/2
  hvs_dcdc_HvCurrent/1 -> Delay/1
  "dcdc_conv_eff vlt, curr, coolantTemp"/1 -> dcdc_conv_eff/1, Product1/1  "dcdc_conv_eff"
  Product2/1 -> Switch/1
  Product1/1 -> Product2/1
  hvs_dcdcConv_current/1 -> Switch/3
  Switch/1 -> hvs_dcdcConv_current1/1  "hvs_dcdcConverter_current"
  dcLink_aux_power/1 -> Product1/2
  Avoid_Div_by_zero/1 -> Product2/2
  Constant/1 -> Switch/2
  hvsAux_dcdcConv_LvVoltage_Rq/1 -> Avoid_Div_by_zero/1
  hvs_dcdcConverter_voltage/1 -> "dcdc_conv_eff vlt, curr, coolantTemp"/1
  hvs_drvEmotCoolant_Temperature/1 -> "dcdc_conv_eff vlt, curr, coolantTemp"/3

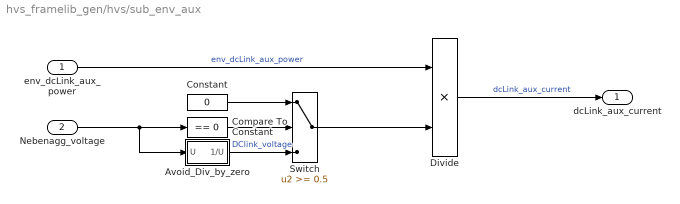
== system hvs_framelib_gen/hvs/sub_env_aux ==
  env_dcLink_aux_power : Inport
  Nebenagg_voltage : Inport  Port=2
  Avoid_Div_by_zero : Subsystem
  Compare To Constant : simulink/Logic and Bit Operations/Compare To Constant  relop===  const=0  OutDataTypeStr=boolean
  Constant : Constant  Value=0
  Divide : Product
  Switch : Switch  Threshold=0.5
  dcLink_aux_current : Outport
  wires:
  Divide/1 -> dcLink_aux_current/1  "dcLink_aux_current"
  Nebenagg_voltage/1 -> Avoid_Div_by_zero/1(U), Compare To Constant/1
  Avoid_Div_by_zero/1(1/U) -> Switch/3  "DClink_voltage"
  env_dcLink_aux_power/1 -> Divide/1  "env_dcLink_aux_power"
  Compare To Constant/1 -> Switch/2
  Constant/1 -> Switch/1
  Switch/1 -> Divide/2

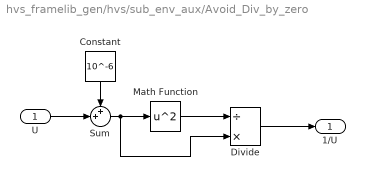
== system hvs_framelib_gen/hvs/sub_env_aux/Avoid_Div_by_zero ==
  U : Inport
  Constant : Constant  Value=10^-6
  Divide : Product  Inputs=/*
  Math Function : Math  Operator=square  SaturateOnIntegerOverflow=on
  Sum : Sum  Inputs=++|
  1/U : Outport
  wires:
  U/1 -> Sum/2
  Constant/1 -> Sum/1
  Sum/1 -> Math Function/1, Divide/2
  Math Function/1 -> Divide/1
  Divide/1 -> 1/U/1
